simulink subsystem "VS_DiscreteTimeModel"  (R2020b)
settings: Solver=VariableStepAuto  StartTime=0.0  StopTime=10.0  RelTol=1e-3
model mask{s0=0, Ts=0, noise_perc=0}
settings Model: Creator=marco  LastModifiedBy=marco

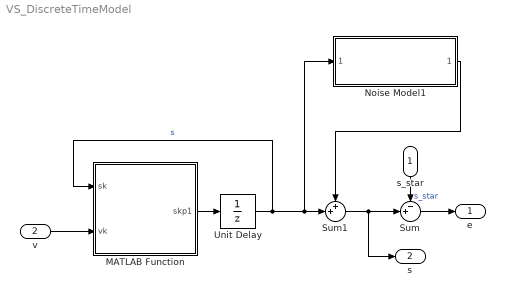
== system VS_DiscreteTimeModel ==
  s_star : Inport
  v : Inport  Port=2
  MATLAB Function : MATLAB Function  TreatAsAtomicUnit=on
  Noise Model1 : Subsystem  ReferencedSubsystem=VSNoiseModel  noise_perc=noise_perc  noise_sample_time=Ts
  Sum : Sum  Inputs=-+|
  Sum1 : Sum  Inputs=++|
  Unit Delay : UnitDelay  InitialCondition=s0  SampleTime=Ts  HasFrameUpgradeWarning=on
  e : Outport
  s : Outport  Port=2
  wires:
  s_star/1 -> Sum/1  "s_star"
  Sum/1 -> e/1
  Noise Model1/1 -> Sum1/1
  Unit Delay/1 -> Sum1/2, Noise Model1/1, MATLAB Function/1(sk)  "s"
  Sum1/1 -> s/1, Sum/2
  MATLAB Function/1(skp1) -> Unit Delay/1
  v/1 -> MATLAB Function/2(vk)

== matlab function VS_DiscreteTimeModel/MATLAB Function ==
  data: sk input; skp1 output; vk input; Ts parameter
function skp1 = fcn(sk, vk,Ts)

skp1 = discreteFeatureSystem(Ts, sk, vk);

%% alternative
% function skp1 = fcn(sk, vk, s_star_k, Ds_star_k, Ts)
% 
% ek = sk - s_star_k;
% 
% ekp1 = discreteErrorSystem(Ts, ek, s_star_k, vk, Ds_star_k);
% 
% s_star_kp1 = Ds_star_k + s_star_k;
% skp1 = ekp1 + s_star_kp1;
